simulink model "Dofbot_Arm"  (R2021b)
settings: Solver=VariableStepAuto  StartTime=0.0  StopTime=10.0  RelTol=1e-3
undefined symbols (not defined in the file or in its folder): X, Y, Z
libraries: sm_lib x60, nesl_utility x16
(part 2 of 2)

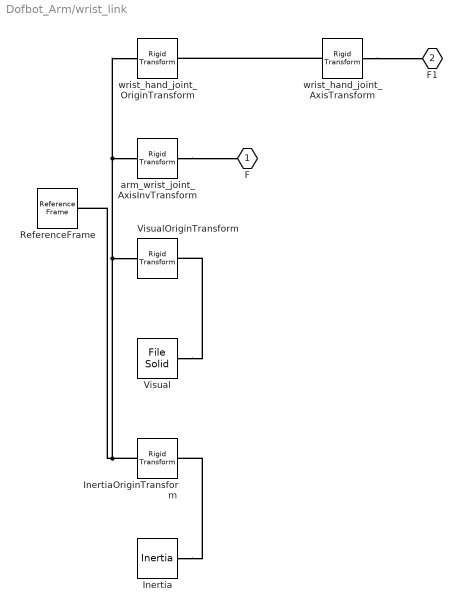
== system Dofbot_Arm/wrist_link ==
  Inertia : sm_lib/Body Elements/Inertia  InertiaType=Custom  Mass=0.04388  MassUnits=kg  CenterOfMass=[0, 0, 0]  CenterOfMassUnits=m  MomentsOfInertia=[1.4107e-05, 1.5344e-05, 9.353200000000001e-06]  MomentsOfInertiaUnits=kg*m^2  ProductsOfInertia=[3.5666e-09, -9.7935e-07, 1.0323e-09]  ProductsOfInertiaUnits=kg*m^2  GraphicType=None  MarkerShape=Inertia  MarkerSize=20  GraphicVisPropType=SimpleVisualProperties  GraphicDiffuseColor=[0.5 0.5 0.5]  GraphicSpecularColor=[0.5 0.5 0.5 1.0]  GraphicAmbientColor=[0.15 0.15 0.15 1.0]  GraphicEmissiveColor=[0.0 0.0 0.0 1.0]  GraphicShininess=75  GraphicOpacity=1.0
  InertiaOriginTransform : sm_lib/Frames and Transforms/Rigid Transform  TranslationMethod=Cartesian  TranslationStandardOffset=0  TranslationLengthUnit=m  TranslationStandardAxis=+Z  TranslationCartesianOffset=[-0.003355, -1.0383e-05, 0.035742]  TranslationROffset=0  TranslationROffsetUnits=m  TranslationZOffset=0  TranslationZOffsetUnits=m  TranslationThetaOffset=0  TranslationThetaOffsetUnits=deg  RotationMethod=RotationSequence  RotationAngleUnits=deg  RotationStandardAxis=+Z  RotationAngle=0.0  RotationArbitraryAxis=[0 0 1]  FollAlignAxisA=+X  BaseAlignAxisA=+Y  FollAlignAxisB=+Y  BaseAlignAxisB=+Z  RotationSequenceAxes=BaseAxes  RotationSequence=XYZ  RotationSequenceAngles=[0, 0, 0]  RotationSequenceAnglesUnits=rad  RotationMatrix=[1 0 0; 0 1 0; 0 0 1]
  ReferenceFrame : sm_lib/Frames and Transforms/Reference Frame
  Visual : sm_lib/Body Elements/File Solid  ExtGeomFileName=D:\Matlab\Dofbot_Arm\meshes\wrist_link.STL  UnitType=Custom  ExtGeomFileUnits=m  StepReaderType=HEX  ExportConvexHullGeometry=off  InertiaType=Custom  Mass=0  MassUnits=kg  CenterOfMass=[0, 0, 0]  CenterOfMassUnits=m  MomentsOfInertia=[0, 0, 0]  MomentsOfInertiaUnits=kg*m^2  ProductsOfInertia=[0, 0, 0]  ProductsOfInertiaUnits=kg*m^2  BasedOnType=DensityFromFile  Density=1000  DensityUnits=kg/m^3  DoExposeReferenceFrame=on  SerializedFrames=<Frames/>  GraphicType=FromGeometry  MarkerShape=Sphere  MarkerSize=10  GraphicVisPropType=SimpleVisualProperties  GraphicDiffuseColor=[0.7529400000000001, 1, 0.7529400000000001]  GraphicSpecularColor=[0.5 0.5 0.5 1.0]  GraphicAmbientColor=[0.15 0.15 0.15 1.0]  GraphicEmissiveColor=[0.0 0.0 0.0 1.0]  GraphicShininess=75  GraphicOpacity=1
  VisualOriginTransform : sm_lib/Frames and Transforms/Rigid Transform  TranslationMethod=Cartesian  TranslationStandardOffset=0  TranslationLengthUnit=m  TranslationStandardAxis=+Z  TranslationCartesianOffset=[0, 0, 0]  TranslationROffset=0  TranslationROffsetUnits=m  TranslationZOffset=0  TranslationZOffsetUnits=m  TranslationThetaOffset=0  TranslationThetaOffsetUnits=deg  RotationMethod=RotationSequence  RotationAngleUnits=deg  RotationStandardAxis=+Z  RotationAngle=0.0  RotationArbitraryAxis=[0 0 1]  FollAlignAxisA=+X  BaseAlignAxisA=+Y  FollAlignAxisB=+Y  BaseAlignAxisB=+Z  RotationSequenceAxes=BaseAxes  RotationSequence=XYZ  RotationSequenceAngles=[0, 0, 0]  RotationSequenceAnglesUnits=rad  RotationMatrix=[1 0 0; 0 1 0; 0 0 1]
  arm_wrist_joint_AxisInvTransform : sm_lib/Frames and Transforms/Rigid Transform  TranslationMethod=Cartesian  TranslationStandardOffset=0  TranslationLengthUnit=m  TranslationStandardAxis=+Z  TranslationCartesianOffset=[0, 0, 0]  TranslationROffset=0  TranslationROffsetUnits=m  TranslationZOffset=0  TranslationZOffsetUnits=m  TranslationThetaOffset=0  TranslationThetaOffsetUnits=deg  RotationMethod=ArbitraryAxis  RotationAngleUnits=rad  RotationStandardAxis=+Z  RotationAngle=1.570796326794897  RotationArbitraryAxis=[-1, 0, 0]  FollAlignAxisA=+X  BaseAlignAxisA=+Y  FollAlignAxisB=+Y  BaseAlignAxisB=+Z  RotationSequenceAxes=FollowerAxes  RotationSequence=XYX  RotationSequenceAngles=[0 0 0]  RotationSequenceAnglesUnits=deg  RotationMatrix=[1 0 0; 0 1 0; 0 0 1]
  wrist_hand_joint_AxisTransform : sm_lib/Frames and Transforms/Rigid Transform  TranslationMethod=Cartesian  TranslationStandardOffset=0  TranslationLengthUnit=m  TranslationStandardAxis=+Z  TranslationCartesianOffset=[0, 0, 0]  TranslationROffset=0  TranslationROffsetUnits=m  TranslationZOffset=0  TranslationZOffsetUnits=m  TranslationThetaOffset=0  TranslationThetaOffsetUnits=deg  RotationMethod=ArbitraryAxis  RotationAngleUnits=rad  RotationStandardAxis=+Z  RotationAngle=0.002064197068171301  RotationArbitraryAxis=[-0, 0.002064195602316829, 0]  FollAlignAxisA=+X  BaseAlignAxisA=+Y  FollAlignAxisB=+Y  BaseAlignAxisB=+Z  RotationSequenceAxes=FollowerAxes  RotationSequence=XYX  RotationSequenceAngles=[0 0 0]  RotationSequenceAnglesUnits=deg  RotationMatrix=[1 0 0; 0 1 0; 0 0 1]
  wrist_hand_joint_OriginTransform : sm_lib/Frames and Transforms/Rigid Transform  TranslationMethod=Cartesian  TranslationStandardOffset=0  TranslationLengthUnit=m  TranslationStandardAxis=+Z  TranslationCartesianOffset=[0.0016634, -4.333e-05, 0.07804899999999999]  TranslationROffset=0  TranslationROffsetUnits=m  TranslationZOffset=0  TranslationZOffsetUnits=m  TranslationThetaOffset=0  TranslationThetaOffsetUnits=deg  RotationMethod=RotationSequence  RotationAngleUnits=deg  RotationStandardAxis=+Z  RotationAngle=0.0  RotationArbitraryAxis=[0 0 1]  FollAlignAxisA=+X  BaseAlignAxisA=+Y  FollAlignAxisB=+Y  BaseAlignAxisB=+Z  RotationSequenceAxes=BaseAxes  RotationSequence=XYZ  RotationSequenceAngles=[0, 0, 0]  RotationSequenceAnglesUnits=rad  RotationMatrix=[1 0 0; 0 1 0; 0 0 1]
  F : PMIOPort  Side=Left
  F1 : PMIOPort  Port=2  Side=Right
  connections:
  Inertia/RConn1 -- InertiaOriginTransform/RConn1
  ReferenceFrame/RConn1 -- InertiaOriginTransform/LConn1 -- arm_wrist_joint_AxisInvTransform/LConn1 -- wrist_hand_joint_OriginTransform/LConn1 -- VisualOriginTransform/LConn1
  Visual/RConn1 -- VisualOriginTransform/RConn1
  arm_wrist_joint_AxisInvTransform/RConn1 -- F/RConn1
  wrist_hand_joint_AxisTransform/RConn1 -- F1/RConn1
  wrist_hand_joint_AxisTransform/LConn1 -- wrist_hand_joint_OriginTransform/RConn1

== matlab function Dofbot_Arm/postura ==
  data: x input; theta_m_1 output; y input; z input; beta input; theta_1_2 output; theta_2_3 output; theta_3_4 output; theta_4_5 output
function [theta_m_1,theta_1_2,theta_2_3,theta_3_4,theta_4_5] = fcn(x,y,z,beta)

%Parametros del robot
%Longitudes de los eslabones
L_1 = 0.08412; %m
L_2 = 0.08412; %m
L_3 = 0.16332; %m

%Componentes del vector p_m_1
%Coordenadas del origen del sistema 1 con respecto al sistema m.
x_m_1 = 0.072;
y_m_1 = 0.0;
z_m_1 = 0.105;

%Definicion de los vectores
p_m_1 = [x_m_1;y_m_1;z_m_1]; %Vector de posicion del sistema 1 con respecto al sistema m
p_m_P = [x;y;z]; % vector de posicion del sistema P con respecto al sistema m

p_1_P = p_m_P-p_m_1;

theta_1_P = atan2(y,(x-x_m_1));
p_P_4 = p_m_P-[L_3*cos(theta_1_P)*cos(beta);L_3*sin(theta_1_P)*cos(beta);L_3*sin(beta)];

p_1_4 = p_1_P+p_P_4;

%Calculo de los angulos complementarios

z_1 = [0;0;1];

Epsilon = acos((dot(z_1,p_1_4))/(norm(z_1)*norm(p_1_4)));
alpha = acos((L_1^2+norm(p_1_4)^2-L_2^2)/(2*L_1*norm(p_1_4)));

beta_r = asin((norm(p_1_4)*sin(alpha))/L_2);

theta_m_1 = atan2(y,(x-x_m_1));
theta_1_2 =Epsilon-alpha;
theta_2_3 = pi-beta_r;
theta_3_4 = beta;
theta_4_5 = 0;

== matlab function Dofbot_Arm/Trayectoria ==
  data: t input; x_P output; y_P output; z_P output; beta_P output
function [x_P,y_P,z_P,beta_P] = fcn(t)

beta_in = 3*pi/4;
beta_fin = 3*pi/4;

t_total = 10; %s

x_in = 0.30; %m
x_fin = 0.30;%m

y_in = 0.15; %m
y_fin = -0.15; %m

z_in = 0.14; %m
z_fin = 0.14; %m

x_P = x_in+((10/t_total^3)*t^3-(15/t_total^4)*t^4+(6/t_total^5)*t^5)*(x_fin-x_in);
y_P = y_in+((10/t_total^3)*t^3-(15/t_total^4)*t^4+(6/t_total^5)*t^5)*(y_fin-y_in);
z_P = z_in+((10/t_total^3)*t^3-(15/t_total^4)*t^4+(6/t_total^5)*t^5)*(z_fin-z_in);
beta_P = beta_in+((10/t_total^3)*t^3-(15/t_total^4)*t^4+(6/t_total^5)*t^5)*(beta_fin-beta_in);
